simulink model "predict"  (R2024b)
settings: Solver=FixedStepAuto  StartTime=0.0  StopTime=10.0  FixedStep=1  RelTol=1e-3
undefined symbols (not defined in the file): A, B, Wk
settings Model: Creator=54238  LastModifiedBy=54238

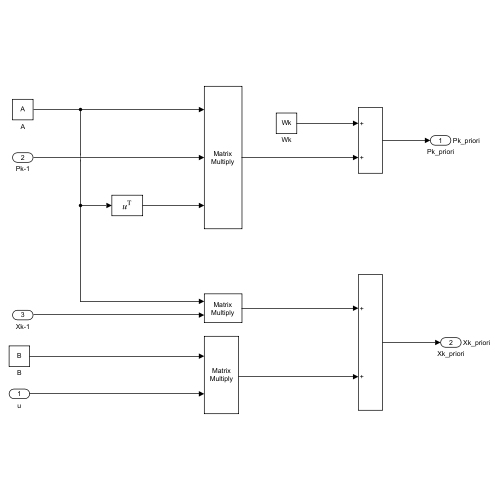
[thumbnail: Simulink's stored preview of the top-level diagram]
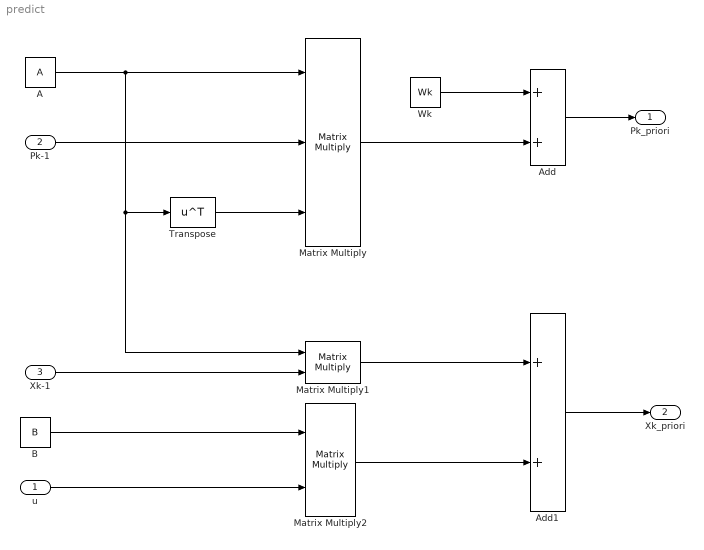
== system predict ==
  u : Inport  PortDimensions=[2,1]
  Pk-1 : Inport  Port=2  PortDimensions=[4,4]
  Xk-1 : Inport  Port=3  PortDimensions=[4,1]
  A : Constant  Value=A
  Add : Sum
  Add1 : Sum
  B : Constant  Value=B
  Matrix Multiply : Product  Inputs=3  Multiplication=Matrix(*)
  Matrix Multiply1 : Product  Multiplication=Matrix(*)
  Matrix Multiply2 : Product  Multiplication=Matrix(*)
  Transpose : Math  Operator=transpose  SignedPower=on  RndMeth=Zero
  Wk : Constant  Value=Wk
  Pk_priori : Outport  SignalName=Pk_priori  PortDimensions=[4,4]
  Xk_priori : Outport  Port=2  SignalName=Xk_priori  PortDimensions=[4,1]
  wires:
  A/1 -> Matrix Multiply1/1, Transpose/1, Matrix Multiply/1
  Pk-1/1 -> Matrix Multiply/2
  Transpose/1 -> Matrix Multiply/3
  u/1 -> Matrix Multiply2/2
  B/1 -> Matrix Multiply2/1
  Matrix Multiply/1 -> Add/2
  Wk/1 -> Add/1
  Add/1 -> Pk_priori/1
  Matrix Multiply1/1 -> Add1/1
  Xk-1/1 -> Matrix Multiply1/2
  Matrix Multiply2/1 -> Add1/2
  Add1/1 -> Xk_priori/1
